simulink model "logs_capture"  (Simulink 7.9)
settings: Solver=FixedStepDiscrete  StartTime=0.0  StopTime=inf  FixedStep=0.01  RelTol=1e-3
undefined symbols (not defined in the file or in its folder): Pbias, Pbias_gyro, Pscale, serial
libraries: instrumentlib x2
settings Model: Creator=root  LastModifiedBy=root
settings DataIOCC: LimitDataPoints=off
settings GRTTargetCC: CodeReplacementLibrary=C99 (ISO)

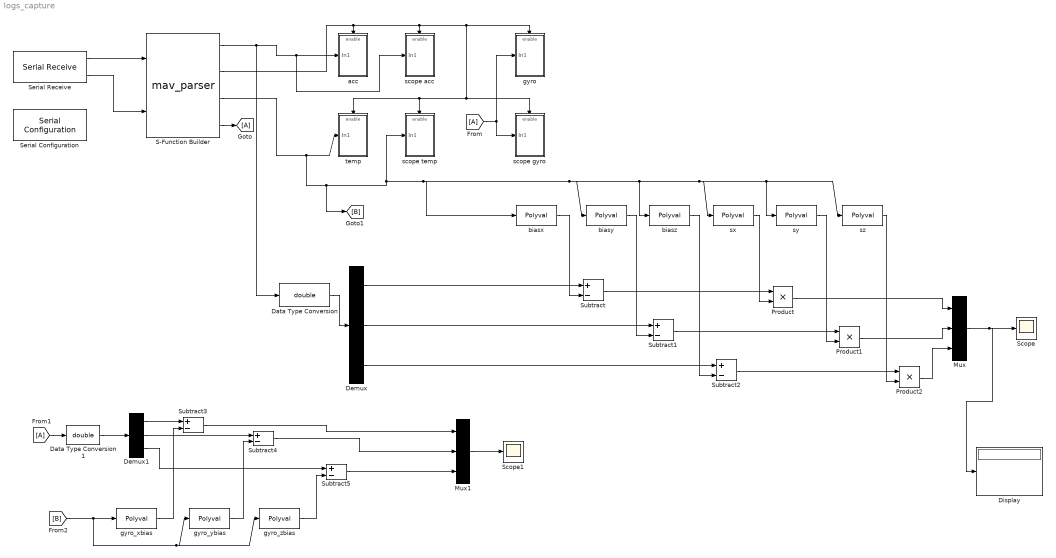
== system logs_capture ==
  Data Type Conversion : DataTypeConversion  OutDataTypeStr=double
  Data Type Conversion1 : DataTypeConversion  OutDataTypeStr=double
  Demux : Demux  Outputs=3
  Demux1 : Demux  Outputs=3
  Display : Display
  Mux : Mux  Inputs=3
  Mux1 : Mux  Inputs=3
  Product : Product  RndMeth=Zero
  Product1 : Product  RndMeth=Zero
  Product2 : Product  RndMeth=Zero
  S-Function Builder : S-Function  InitFcn=try, set_param(gcb,'FunctionName','mav_parser'), end  FunctionName=mav_parser  SFunctionModules=mav_parser_wrapper  WizardData=DataTag0  EnableBusSupport=off  mask(S-Function Builder){}
      mask help: Simulink:masks:SFunctionBuilder_MD
      mask init:
      | val = [[.9  0.75 0.75 1 1 .9 .9 1]',[1 1 0.75 0.75 .9 .9 1 .9]'];try , sys = get_param(gcb,'SfunBuilderFcnName');if isempty(sys), sys = get_param(gcb,'FunctionName'); end,catch, sys = get_param(gcb,'FunctionName'); end
      settings: CopyFcn=set_param(gcbh,'LinkStatus','none')  PreSaveFcn=try, set_param(gcb,'FunctionName','mav_parser'), end  OpenFcn=sfunctionwizard(gcbh)
      mask Display: plot(val(:,1),val(:,2)),disp(sys), port_label('input',1,'uart_byte'), port_label('input',2,'uart_status'), port_label('output',1,'acc'), port_label('output',2,'imu_en'), port_label('output',3,'temp'), port_label('output',4,'gyro')
  Scope : Scope
      settings: TimeRange=5000  YMin=-12000  YMax=12000
  Scope1 : Scope
      settings: TimeRange=1000  YMin=-100  YMax=100  SaveName=ScopeData2
  Serial Configuration : instrumentlib/Serial Configuration  Priority=-200000  ComPortMenu=/dev/ttyS64  ComPort=/dev/ttyS64  ObjConstructor=serial('/dev/ttyS64');  BaudRate=115200  DataBits=8  Parity=none  StopBits=1  FlowControl=none  Timeout=10  ByteOrder=LittleEndian
  Serial Receive : instrumentlib/Serial Receive  ComPortMenu=/dev/ttyS64  ComPort=/dev/ttyS64  ObjConstructor=serial('/dev/ttyS64');  Terminator=<none>  DataSize="[256    1]"  DataType=uint8  EnableBlockingMode=off  ActionDataUnavailable=Output last received value  CustomValue=0  SampleTime=0.01
  Subtract{,1..5} (6 alike) : Sum  Inputs=+-
  acc : Subsystem
  biasx : Polyval  Coefs=Pbias(1,:)
  biasy : Polyval  Coefs=Pbias(2,:)
  biasz : Polyval  Coefs=Pbias(3,:)
  gyro : Subsystem
  gyro_xbias : Polyval  Coefs=Pbias_gyro(1,:)
  gyro_ybias : Polyval  Coefs=Pbias_gyro(2,:)
  gyro_zbias : Polyval  Coefs=Pbias_gyro(3,:)
  scope acc : Subsystem
  scope gyro : Subsystem
  scope temp : Subsystem
  sx : Polyval  Coefs=Pscale(1,:)
  sy : Polyval  Coefs=Pscale(2,:)
  sz : Polyval  Coefs=Pscale(3,:)
  temp : Subsystem
  wires:
  Serial Receive/1 -> S-Function Builder/1
  Serial Receive/2 -> S-Function Builder/2
  S-Function Builder/1 -> acc/1(In1), scope acc/1(In1), Data Type Conversion/1
  S-Function Builder/3 -> temp/1(In1), scope temp/1(In1), biasx/1, biasy/1, biasz/1, sx/1, sy/1, sz/1, [B]
  S-Function Builder/2 -> acc/Enable, scope acc/Enable, gyro/Enable, scope temp/Enable, temp/Enable, scope gyro/Enable
  Data Type Conversion/1 -> Demux/1
  Demux/1 -> Subtract/1
  Demux/2 -> Subtract1/1
  Demux/3 -> Subtract2/1
  biasx/1 -> Subtract/2
  biasy/1 -> Subtract1/2
  biasz/1 -> Subtract2/2
  Subtract/1 -> Product/1
  Subtract1/1 -> Product1/1
  sx/1 -> Product/2
  sy/1 -> Product1/2
  Subtract2/1 -> Product2/1
  sz/1 -> Product2/2
  Product/1 -> Mux/1
  Product1/1 -> Mux/2
  Product2/1 -> Mux/3
  Mux/1 -> Scope/1, Display/1
  S-Function Builder/4 -> [A]
  [A] -> scope gyro/1(In1), gyro/1(In1)
  [A] -> Data Type Conversion1/1
  Data Type Conversion1/1 -> Demux1/1
  Demux1/1 -> Subtract3/1
  Demux1/2 -> Subtract4/1
  Subtract3/1 -> Mux1/1
  Subtract4/1 -> Mux1/2
  Subtract5/1 -> Mux1/3
  gyro_xbias/1 -> Subtract3/2
  gyro_ybias/1 -> Subtract4/2
  gyro_zbias/1 -> Subtract5/2
  [B] -> gyro_xbias/1, gyro_ybias/1, gyro_zbias/1
  Mux1/1 -> Scope1/1
  Demux1/3 -> Subtract5/1

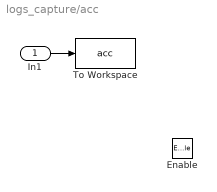
== system logs_capture/acc ==
  In1 : Inport
  Enable : EnablePort
  To Workspace : ToWorkspace  VariableName=acc  SampleTime=-1
  wires:
  In1/1 -> To Workspace/1

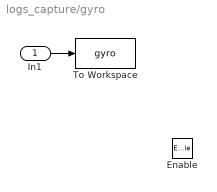
== system logs_capture/gyro ==
  In1 : Inport
  Enable : EnablePort
  To Workspace : ToWorkspace  VariableName=gyro  SampleTime=-1
  wires:
  In1/1 -> To Workspace/1

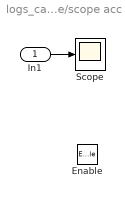
== system logs_capture/scope acc ==
  In1 : Inport
  Enable : EnablePort
  Scope : Scope
      settings: TimeRange=5000  YMin=-500  YMax=10000
  wires:
  In1/1 -> Scope/1

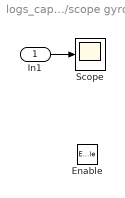
== system logs_capture/scope gyro ==
  In1 : Inport
  Enable : EnablePort
  Scope : Scope
      settings: TimeRange=1000  YMin=-100  YMax=100
  wires:
  In1/1 -> Scope/1

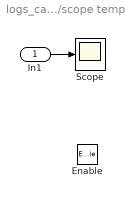
== system logs_capture/scope temp ==
  In1 : Inport
  Enable : EnablePort
  Scope : Scope
      settings: TimeRange=5000  YMin=30  YMax=80
  wires:
  In1/1 -> Scope/1

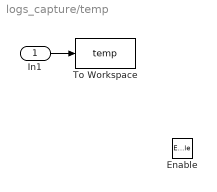
== system logs_capture/temp ==
  In1 : Inport
  Enable : EnablePort
  To Workspace : ToWorkspace  VariableName=temp  SampleTime=-1
  wires:
  In1/1 -> To Workspace/1
